simulink model "ThreeTankRT"  (R2022b)
settings: Solver=ode5  StartTime=0.0  StopTime=200  FixedStep=0.1  RelTol=1e-3  EnableMultiTasking=on
values from neighbouring files (symbols this model uses):
  H1 = [-1.351351351351351e+02,6.689189189189188e+02]    [Initialise_MiniThreetank_System_A.m]    (also in Initialise_MiniThreetank_System_C.m = [-1.334044823906083e+02,6.681963713980788e+02]; Initialise_MiniThreetank_System_D.m = [-1.334757074212494e+02,6.618526428190070e+02]; Initialise_MiniThreetank_System_H.m = [-1.363636363636364e+02,6.584545454545455e+02])
  H2 = [-1.344086021505376e+02,6.588709677419354e+02]    [Initialise_MiniThreetank_System_A.m]    (also in Initialise_MiniThreetank_System_C.m = [-1.335470085470086e+02,6.647168803418803e+02]; Initialise_MiniThreetank_System_D.m = [-1.341201716738198e+02,6.680257510729615e+02]; Initialise_MiniThreetank_System_H.m = [-1.359434475258292e+02,6.459760739532353e+02])
  H3 = [-1.351351351351351e+02,6.513513513513514e+02]    [Initialise_MiniThreetank_System_A.m]    (also in Initialise_MiniThreetank_System_C.m = [-1.334396597554492e+02,6.671584263689527e+02]; Initialise_MiniThreetank_System_D.m = [-1.346566523605150e+02,6.562242489270387e+02]; Initialise_MiniThreetank_System_H.m = [-1.346257404415725e+02,6.457189014539581e+02])
  P1 = [0,5.435299228977511]    [Initialise_MiniThreetank_System_A.m]    (also in Initialise_MiniThreetank_System_C.m = [0,4.885840481157109]; Initialise_MiniThreetank_System_D.m = [0,4.758272391648974]; Initialise_MiniThreetank_System_H.m = [0,4.483707856844433])
  P2 = [0,4.997863989252405]    [Initialise_MiniThreetank_System_A.m]    (also in Initialise_MiniThreetank_System_C.m = [0,5.089076298275632]; Initialise_MiniThreetank_System_D.m = [0,4.950856816941413]; Initialise_MiniThreetank_System_H.m = [0,4.655506526469390])
  Qlimit = 20    [Initialise_MiniThreetank_System_A.m]    (also in Initialise_MiniThreetank_System_C.m; Initialise_MiniThreetank_System_D.m; Initialise_MiniThreetank_System_H.m)
undefined symbols (not defined in the file or in its folder): Serial_Port, Standard_Devices
libraries: hilink x5
settings Model: ModifiedByFormat=C. Gokcek  SimulationMode=external  ExtModeTrigDuration=20480  Creator=C. Gokcek  LastModifiedBy=C. Gokcek
settings SolverCC: AlgebraicLoopSolver=TrustRegion
settings DataIOCC: SaveFormat=Array  SaveOutput=off  SignalLogging=off  DSMLogging=off  SaveTime=off  ReturnWorkspaceOutputs=off
settings OptimizationCC: ExpressionDepthLimit=2147483647  InitFltsAndDblsToZero=on  EfficientMapNaN2IntZero=off  LifeSpan=inf  SimCompilerOptimization=on
settings DebuggingCC: UnderspecifiedInitializationDetection=Classic  MergeDetectMultiDrivingBlocksExec=none  UnconnectedInputMsg=warning  UnconnectedOutputMsg=warning  UnconnectedLineMsg=warning  AllowSymbolicDim=off  StateNameClashWarn=warning  SFUnexpectedBacktrackingDiag=warning  SFNoUnconditionalDefaultTransitionDiag=warning  SFExecutionAtInitializationDiag=none  SFMachineParentedDataDiag=warning  ArithmeticOperatorsInVariantConditions=warning
settings HardwareCC: ProdBitPerLong=64  ProdHWDeviceType=Intel->x86-64 (Linux 64)  TargetBitPerLong=64  TargetBitPerPointer=64  TargetIntDivRoundTo=Zero  TargetEndianess=LittleEndian  TargetWordSize=64  TargetHWDeviceType=Intel->x86-64
settings ModelReferenceCC: EnableRefExpFcnMdlSchedulingChecks=on  PropagateSignalLabelsOutOfModel=off
settings SFSimCC: SimUseLocalCustomCode=off  CustomCodeUndefinedFunction=UseInterfaceOnly
settings RTWCC: Description=Simulink Desktop Real-Time  SystemTargetFile=sldrt.tlc  TemplateMakefile=sldrt.tmf  RTWVerbose=off  TLCAssert=on  RTWUseLocalCustomCode=off  RTWCompilerOptimization=on  DLArmComputeVersion=19.05
settings CodeAppCC: GenerateComments=off  MaxIdLength=95  SimulinkBlockComments=off
settings SimulinkDesktopRealTimeCC: TargetLibSuffix=_sldrt.a  TargetPreCompLibLocation=C:\Program Files\MATLAB\R2022b\toolbox\sldrt\lib\win64  TargetLangStandard=C89/C90 (ANSI)  SupportVariableSizeSignals=off
settings ConfigComp: CovMetricSettings=dw  CovSaveCumulativeToWorkspaceVar=on  CovSaveSingleToWorkspaceVar=on  CovExternalEMLEnable=off  CovSFcnEnable=off

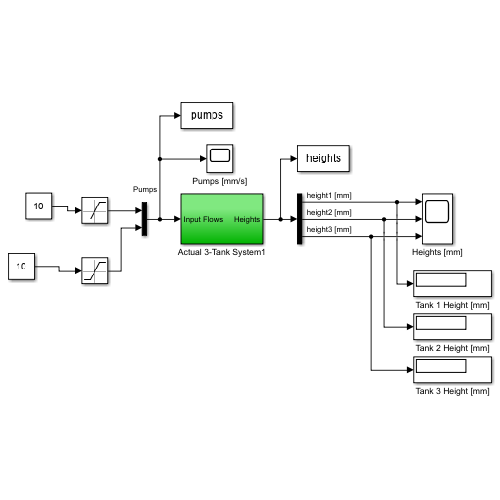
[thumbnail: Simulink's stored preview of the top-level diagram]
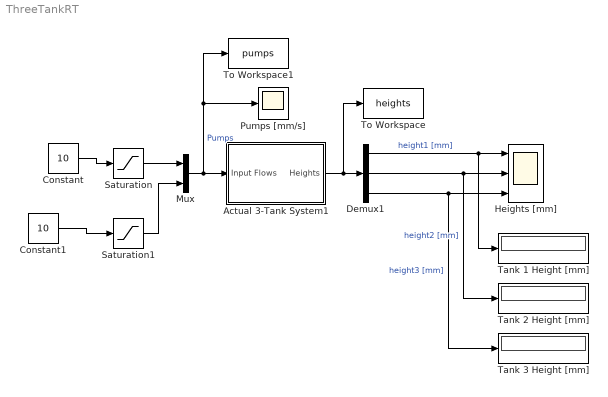
== system ThreeTankRT ==
  Actual 3-Tank System1 : Subsystem
  Constant : Constant  Value=10
  Constant1 : Constant  Value=10
  Demux1 : Demux  Outputs=3
  Heights [mm] : Scope  NumInputPorts=3
  Mux : Mux  Inputs=2
  Pumps [mm/s] : Scope
  Saturation : Saturate  UpperLimit=Qlimit  LowerLimit=0  LinearizeAsGain=off
  Saturation1 : Saturate  UpperLimit=Qlimit  LowerLimit=0  LinearizeAsGain=off
  Tank 1 Height [mm] : Display
  Tank 2 Height [mm] : Display
  Tank 3 Height [mm] : Display
  To Workspace : ToWorkspace  VariableName=heights  SaveFormat=Structure With Time  SampleTime=-1
  To Workspace1 : ToWorkspace  VariableName=pumps  SaveFormat=Structure With Time  SampleTime=-1
  wires:
  Actual 3-Tank System1/1(Heights) -> To Workspace/1, Demux1/1
  Demux1/3 -> Tank 3 Height [mm]/1, Heights [mm]/3  "height3 [mm]"
  Demux1/1 -> Tank 1 Height [mm]/1, Heights [mm]/1  "height1 [mm]"
  Demux1/2 -> Tank 2 Height [mm]/1, Heights [mm]/2  "height2 [mm]"
  Mux/1 -> Actual 3-Tank System1/1(Input Flows), Pumps [mm/s]/1, To Workspace1/1  "Pumps"
  Saturation/1 -> Mux/1
  Saturation1/1 -> Mux/2
  Constant/1 -> Saturation/1
  Constant1/1 -> Saturation1/1

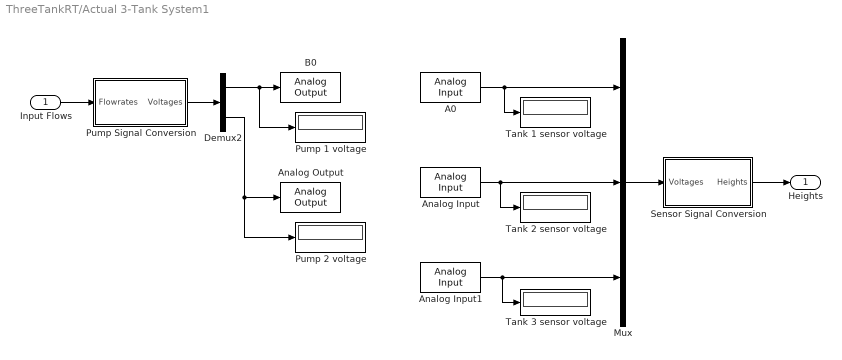
== system ThreeTankRT/Actual 3-Tank System1 ==
  Input Flows : Inport
  A0 : hilink/Analog Input  SampleTime=0.1  MaxMissedTicks=10  ShowMissedTicks=0  YieldWhenWaiting=0  DrvName=Standard_Devices/Serial_Port  DrvAddress=1  DrvOptions=[115200 8 0 0 0 0 0 0]  PacketSize=8  DataTypes='double'  ShowReady=0  ShowError=0  PacketID=1  ByteOrder=1  ShowTimestamp=0  CfgPrm=A0  PrmCfg=unipolar  ResVar=0  VarRes=0
      settings: SourceProductName=Hilink
  Analog Input : hilink/Analog Input  SampleTime=0.1  MaxMissedTicks=10  ShowMissedTicks=0  YieldWhenWaiting=0  DrvName=Standard_Devices/Serial_Port  DrvAddress=1  DrvOptions=[115200 8 0 0 0 0 0 0]  PacketSize=8  DataTypes='double'  ShowReady=0  ShowError=0  PacketID=1  ByteOrder=1  ShowTimestamp=0  CfgPrm=A1  PrmCfg=unipolar  ResVar=0  VarRes=0
      settings: SourceProductName=Hilink
  Analog Input1 : hilink/Analog Input  SampleTime=0.1  MaxMissedTicks=10  ShowMissedTicks=0  YieldWhenWaiting=0  DrvName=Standard_Devices/Serial_Port  DrvAddress=1  DrvOptions=[115200 8 0 0 0 0 0 0]  PacketSize=8  DataTypes='double'  ShowReady=0  ShowError=0  PacketID=1  ByteOrder=1  ShowTimestamp=0  CfgPrm=A2  PrmCfg=unipolar  ResVar=0  VarRes=0
      settings: SourceProductName=Hilink
  Analog Output : hilink/Analog Output  SampleTime=0.1  MaxMissedTicks=10  ShowMissedTicks=0  YieldWhenWaiting=0  DrvName=Standard_Devices/Serial_Port  DrvAddress=1  DrvOptions=[115200 8 0 0 0 0 0 0]  PacketSize=8  DataTypes='double'  ShowReady=0  ShowError=0  PacketID=1  ByteOrder=1  InitialValue=0  FinalValue=0  CfgPrm=B1  PrmCfg=unipolar  ResVar=0  VarRes=0
      settings: SourceProductName=Hilink
  B0 : hilink/Analog Output  SampleTime=0.1  MaxMissedTicks=10  ShowMissedTicks=0  YieldWhenWaiting=0  DrvName=Standard_Devices/Serial_Port  DrvAddress=1  DrvOptions=[115200 8 0 0 0 0 0 0]  PacketSize=8  DataTypes='double'  ShowReady=0  ShowError=0  PacketID=1  ByteOrder=1  InitialValue=0  FinalValue=0  CfgPrm=B0  PrmCfg=unipolar  ResVar=0  VarRes=0
      settings: SourceProductName=Hilink
  Demux2 : Demux  Outputs=2
  Mux : Mux  Inputs=3
  Pump 1 voltage : Display
  Pump 2 voltage : Display
  Pump Signal Conversion : Subsystem
  "Sensor Signal Conversion " : Subsystem
  Tank 1 sensor voltage : Display
  Tank 2 sensor voltage : Display
  Tank 3 sensor voltage : Display
  Heights : Outport  VectorParamsAs1DForOutWhenUnconnected=off
  wires:
  Pump Signal Conversion/1(Voltages) -> Demux2/1
  Mux/1 -> "Sensor Signal Conversion "/1(Voltages)
  Input Flows/1 -> Pump Signal Conversion/1(Flowrates)
  "Sensor Signal Conversion "/1(Heights) -> Heights/1
  A0/1 -> Tank 1 sensor voltage/1, Mux/1
  Analog Input/1 -> Tank 2 sensor voltage/1, Mux/2
  Demux2/2 -> Pump 2 voltage/1, Analog Output/1
  Analog Input1/1 -> Tank 3 sensor voltage/1, Mux/3
  Demux2/1 -> Pump 1 voltage/1, B0/1

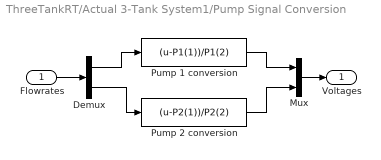
== system ThreeTankRT/Actual 3-Tank System1/Pump Signal Conversion ==
  Flowrates : Inport
  Demux : Demux  Outputs=2
      settings: DisplayOption=none
  Mux : Mux  Inputs=2
  Pump 1 conversion : Fcn  Expr=(u-P1(1))/P1(2)
  Pump 2 conversion : Fcn  Expr=(u-P2(1))/P2(2)
  Voltages : Outport  VectorParamsAs1DForOutWhenUnconnected=off
  wires:
  Mux/1 -> Voltages/1
  Pump 1 conversion/1 -> Mux/1
  Pump 2 conversion/1 -> Mux/2
  Flowrates/1 -> Demux/1
  Demux/1 -> Pump 1 conversion/1
  Demux/2 -> Pump 2 conversion/1

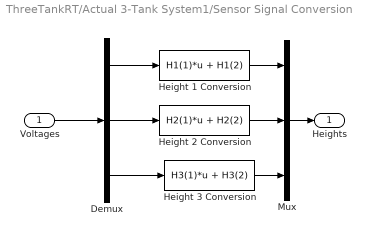
== system ThreeTankRT/Actual 3-Tank System1/Sensor Signal Conversion  ==
  Voltages : Inport
  Demux : Demux  Outputs=3
      settings: DisplayOption=none
  Height 1 Conversion : Fcn  Expr=H1(1)*u + H1(2)
  Height 2 Conversion : Fcn  Expr=H2(1)*u + H2(2)
  Height 3 Conversion : Fcn  Expr=H3(1)*u + H3(2)
  Mux : Mux  Inputs=3
  Heights : Outport  VectorParamsAs1DForOutWhenUnconnected=off
  wires:
  Voltages/1 -> Demux/1
  Demux/1 -> Height 1 Conversion/1
  Demux/2 -> Height 2 Conversion/1
  Demux/3 -> Height 3 Conversion/1
  Height 1 Conversion/1 -> Mux/1
  Height 2 Conversion/1 -> Mux/2
  Height 3 Conversion/1 -> Mux/3
  Mux/1 -> Heights/1
